simulink model "OnBoardMatlabExpo3"  (R2015b)
settings: Solver=FixedStepDiscrete  SolverMode=SingleTasking  StartTime=0.0  StopTime=10.0  FixedStep=0.002  RelTol=1e-3
PreLoadFcn:
  | waijung.modelPreload; % Required for working with Waijung Blockset. Do not remove.
undefined symbols (not defined in the file): CPHA_1Edge, CPOL_Low, Duplex, FirstBit_MSB, Full, Link, LQFP100, ST, STM32F407VG, STM32F4DISCOVERY
libraries: simulink x12, stm32f4_io_lib x7, cube_lib x3, stm32f4_spi_lib x3, stm32f4_device_config_lib x1, BC_USB x1, stm32f4_adc_lib x1
(part 2 of 2)

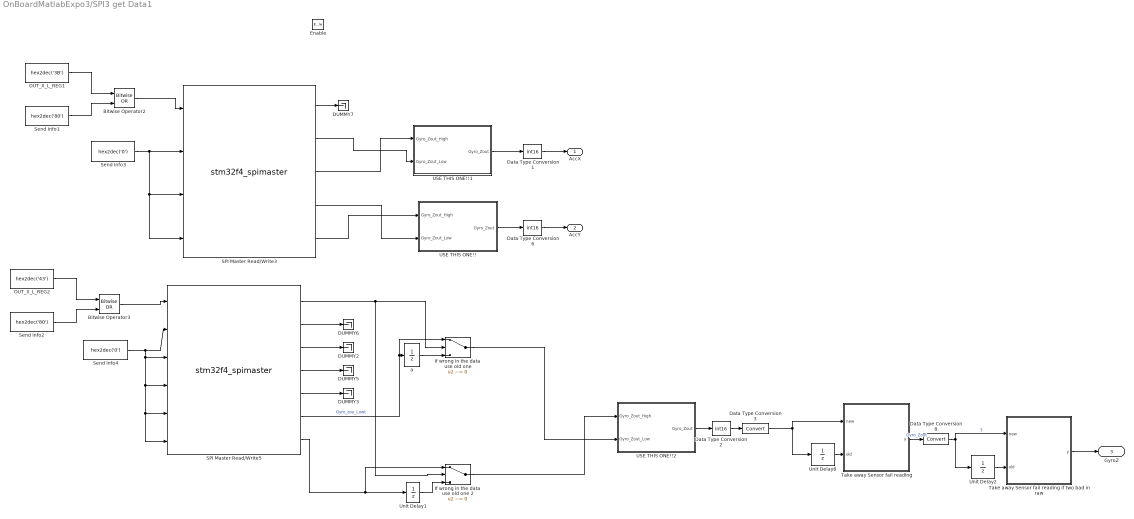
== system OnBoardMatlabExpo3/SPI3 get Data1 ==
  Enable : EnablePort
  " a" : UnitDelay  SampleTime=-1
  Bitwise Operator2 : simulink/Logic and Bit Operations/Bitwise Operator  logicop=OR  UseBitMask=off  NumInputPorts=2  BitMask=bin2dec('11011001')  BitMaskRealWorld=Stored Integer
  Bitwise Operator3 : simulink/Logic and Bit Operations/Bitwise Operator  logicop=OR  UseBitMask=off  NumInputPorts=2  BitMask=bin2dec('11011001')  BitMaskRealWorld=Stored Integer
  DUMMY{2..3,5..7} (5 alike) : Terminator
  Data Type Conversion1 : DataTypeConversion  OutDataTypeStr=int16
  Data Type Conversion2 : DataTypeConversion  OutDataTypeStr=int16
  Data Type Conversion3 : DataTypeConversion
  Data Type Conversion6 : DataTypeConversion  OutDataTypeStr=int16
  Data Type Conversion8 : DataTypeConversion
  If wrong in the data use old one : Switch  Criteria=u2 ~= 0
  If wrong in the data use old one 2 : Switch  Criteria=u2 ~= 0
  OUT_X_L_REG1 : Constant  Value=hex2dec('3B')  OutDataTypeStr=uint8
  OUT_X_L_REG2 : Constant  Value=hex2dec('43')  OutDataTypeStr=uint8
  SPI Master Read/Write3 : S-Function  FunctionName=stm32f4_spimaster  Parameters=mode,configuration,module,datacount,inputtypearray,outputtypearray,confstr,sampletime,sampletimestr,blockid  SFunctionDeploymentMode=off  EnableBusSupport=off  mask(stm32f4_spimaster){configuration=Transaction, module=3, mode=Read/ Write, lastmodule=1, direction=Full-Duplex, dataformat=8bit/ FirstBit_MSB, prescaler=4, cpolcpha=CPOL_Low/ CPHA_1Edge, datacount=4, nssmode=Custom, nsspin=Not used, softnssport=E, softnsspin=0, sckpin=A5, misopin=A6, mosipin=A7, inputtypearray=[4 3 3 3 3], outputtypearray=[5 7 3 3 3 3], confstr=["SPI_Direction_2Lines_FullDuplex","8b","MSB","Low","1Edge","4","Soft","0","x","x","0","x","x","1","A","5","1","A","6","1","A","7","1","0","0","0","0","0","0","0","0","PP","0","UP"], sampletime=-1, sampletimestr=Inf, blockid=SPI3getData1SPIMasterReadWrite3}
      mask prompts: module "SPI Module:"; lastmodule "Last module:"; dataformat "Data format:"; prescaler "Buad rate prescaler: Pclk/"; cpolcpha "Clock polarity (CPOL)/ Clock phase (CPHA):"; datacount "Data Read/Write count:"; nssmode "Slave/chip select (nSS, nCS) mode"; nsspin "Slave/chip select (nSS, nCS) pin"; softnssport "Slave/chip select port (nSS, nCS)"; softnsspin "Slave/chip select pin (nSS, nCS)"; sckpin "SCLK pin:"; misopin "MISO pin:"; mosipin "MOSI pin:"; inputtypearray "Input type array"; outputtypearray "Output type array"; confstr "Configuration string"; sampletime "Sample time (sec)"; sampletimestr "Compiled sample time (sec) in string"
      mask help:
      | Status:
      |  0 - Success.
      |  Otherwise - Fail.
      mask init:
      | stm32f4_spimaster_callback('init');
      mask Help: web(fullfile(waijungdocroot,'stm32f4_spimaster_readwrite.htm'), '-browser')
      mask TypeOptions configuration: Setup | Transaction
      mask Callback configuration: stm32f4_spimaster_callback('configuration');
      mask TypeOptions module: 1 | 2 | 3
      mask Callback module: stm32f4_spimaster_callback('module');
      mask TypeOptions mode: Read/ Write | Read | Write
      mask Callback mode: stm32f4_spimaster_callback('mode');
      mask TypeOptions direction: Full-Duplex | Half-Duplex_Tx | Half-Duplex_Rx
      mask Callback direction: stm32f4_spimaster_callback('direction');
      mask TypeOptions dataformat: 8bit/ FirstBit_MSB | 8bit/ FirstBit_LSB | 16bit/ FirstBit_MSB | 16bit/ FirstBit_LSB
      mask TypeOptions prescaler: 2 | 4 | 8 | 16 | 32 | 64 | 128 | 256
      mask TypeOptions cpolcpha: CPOL_Low/ CPHA_1Edge | CPOL_Low/ CPHA_2Edge | CPOL_High/ CPHA_1Edge | CPOL_High/ CPHA_2Edge
      mask Callback datacount: stm32f4_spimaster_callback('datacount');
      mask TypeOptions nssmode: Hardware | Software | Custom
      mask Callback nssmode: stm32f4_spimaster_callback('nssmode');
      mask TypeOptions nsspin: Not used | A4 | A15
      mask TypeOptions softnssport: A | B | C | D | E | F | G | H | I
      mask TypeOptions softnsspin: 0 | 1 | 2 | 3 | 4 | 5 | 6 | 7 | 8 | 9 | 10 | 11 | 12 | 13 | 14 | 15
      mask TypeOptions sckpin: Not used | A5 | B3
      mask TypeOptions misopin: Not used | A6 | B4
      mask TypeOptions mosipin: Not used | A7 | B5
      mask Callback confstr: stm32f4_spimaster_callback('confstr');
      mask Callback sampletime: stm32f4_spimaster_callback('sampletime');
      mask Callback sampletimestr: stm32f4_spimaster_callback('sampletimestr');
      mask Callback blockid: stm32f4_spimaster_callback('blockid');
      mask Display: text(0.5, 0.5, 'Module: SPI3 (Master)\nRead/ Write\nTs (sec): Inf','ver','middle','hor','center');port_label('input', 1,'Wr0 (uint8)');port_label('input', 2,'Wr1 (uint8)');port_label('input', 3,'Wr2 (uint8)');port_label('input', 4,'Wr3 (uint8)');port_label('output', 1,'Status');port_label('output', 2,'Rd0 (uint8)');port_label('output', 3,'Rd1 (uint8)');port_label('output', 4,'Rd2 (uint8)');port_label('output', 5,'Rd3 (uint8)');
  SPI Master Read/Write5 : S-Function  FunctionName=stm32f4_spimaster  Parameters=mode,configuration,module,datacount,inputtypearray,outputtypearray,confstr,sampletime,sampletimestr,blockid  SFunctionDeploymentMode=off  EnableBusSupport=off  mask(stm32f4_spimaster){configuration=Transaction, module=3, mode=Read/ Write, lastmodule=1, direction=Full-Duplex, dataformat=8bit/ FirstBit_MSB, prescaler=4, cpolcpha=CPOL_Low/ CPHA_1Edge, datacount=6, nssmode=Custom, nsspin=Not used, softnssport=E, softnsspin=0, sckpin=A5, misopin=A6, mosipin=A7, inputtypearray=[6 3 3 3 3 3 3], outputtypearray=[7 7 3 3 3 3 3 3], confstr=["SPI_Direction_2Lines_FullDuplex","8b","MSB","Low","1Edge","4","Soft","0","x","x","0","x","x","1","A","5","1","A","6","1","A","7","1","0","0","0","0","0","0","0","0","PP","0","UP"], sampletime=-1, sampletimestr=Inf, blockid=SPI3getData1SPIMasterReadWrite5}
      mask prompts: module "SPI Module:"; lastmodule "Last module:"; dataformat "Data format:"; prescaler "Buad rate prescaler: Pclk/"; cpolcpha "Clock polarity (CPOL)/ Clock phase (CPHA):"; datacount "Data Read/Write count:"; nssmode "Slave/chip select (nSS, nCS) mode"; nsspin "Slave/chip select (nSS, nCS) pin"; softnssport "Slave/chip select port (nSS, nCS)"; softnsspin "Slave/chip select pin (nSS, nCS)"; sckpin "SCLK pin:"; misopin "MISO pin:"; mosipin "MOSI pin:"; inputtypearray "Input type array"; outputtypearray "Output type array"; confstr "Configuration string"; sampletime "Sample time (sec)"; sampletimestr "Compiled sample time (sec) in string"
      mask help:
      | Status:
      |  0 - Success.
      |  Otherwise - Fail.
      mask init:
      | stm32f4_spimaster_callback('init');
      mask Help: web(fullfile(waijungdocroot,'stm32f4_spimaster_readwrite.htm'), '-browser')
      mask TypeOptions configuration: Setup | Transaction
      mask Callback configuration: stm32f4_spimaster_callback('configuration');
      mask TypeOptions module: 1 | 2 | 3
      mask Callback module: stm32f4_spimaster_callback('module');
      mask TypeOptions mode: Read/ Write | Read | Write
      mask Callback mode: stm32f4_spimaster_callback('mode');
      mask TypeOptions direction: Full-Duplex | Half-Duplex_Tx | Half-Duplex_Rx
      mask Callback direction: stm32f4_spimaster_callback('direction');
      mask TypeOptions dataformat: 8bit/ FirstBit_MSB | 8bit/ FirstBit_LSB | 16bit/ FirstBit_MSB | 16bit/ FirstBit_LSB
      mask TypeOptions prescaler: 2 | 4 | 8 | 16 | 32 | 64 | 128 | 256
      mask TypeOptions cpolcpha: CPOL_Low/ CPHA_1Edge | CPOL_Low/ CPHA_2Edge | CPOL_High/ CPHA_1Edge | CPOL_High/ CPHA_2Edge
      mask Callback datacount: stm32f4_spimaster_callback('datacount');
      mask TypeOptions nssmode: Hardware | Software | Custom
      mask Callback nssmode: stm32f4_spimaster_callback('nssmode');
      mask TypeOptions nsspin: Not used | A4 | A15
      mask TypeOptions softnssport: A | B | C | D | E | F | G | H | I
      mask TypeOptions softnsspin: 0 | 1 | 2 | 3 | 4 | 5 | 6 | 7 | 8 | 9 | 10 | 11 | 12 | 13 | 14 | 15
      mask TypeOptions sckpin: Not used | A5 | B3
      mask TypeOptions misopin: Not used | A6 | B4
      mask TypeOptions mosipin: Not used | A7 | B5
      mask Callback confstr: stm32f4_spimaster_callback('confstr');
      mask Callback sampletime: stm32f4_spimaster_callback('sampletime');
      mask Callback sampletimestr: stm32f4_spimaster_callback('sampletimestr');
      mask Callback blockid: stm32f4_spimaster_callback('blockid');
      mask Display: text(0.5, 0.5, 'Module: SPI3 (Master)\nRead/ Write\nTs (sec): Inf','ver','middle','hor','center');port_label('input', 1,'Wr0 (uint8)');port_label('input', 2,'Wr1 (uint8)');port_label('input', 3,'Wr2 (uint8)');port_label('input', 4,'Wr3 (uint8)');port_label('input', 5,'Wr4 (uint8)');port_label('input', 6,'Wr5 (uint8)');port_label('output', 1,'Status');port_label('output', 2,'Rd0 (uint8)');port_label('output', 3,'Rd1 (uint8)');port_label('output', 4,'Rd2 (uint8)');port_label('output', 5,'Rd3 (uint8)');port_label('output', 6,'Rd4 (uint8)');port_label('output', 7,'Rd5 (uint8)');
  Send Info1 : Constant  Value=hex2dec('80')  OutDataTypeStr=uint8
  Send Info2 : Constant  Value=hex2dec('80')  OutDataTypeStr=uint8
  Send Info3 : Constant  Value=hex2dec('0')  OutDataTypeStr=uint8
  Send Info4 : Constant  Value=hex2dec('0')  OutDataTypeStr=uint8
  Take away Sensor fail reading : MATLAB Function  TreatAsAtomicUnit=on
  Take away Sensor fail reading if two bad in raw : MATLAB Function  TreatAsAtomicUnit=on
  USE THIS ONE!! : Subsystem
  USE THIS ONE!!1 : Subsystem
  USE THIS ONE!!2 : Subsystem
  Unit Delay1 : UnitDelay  SampleTime=-1
  Unit Delay2 : UnitDelay  InitialCondition=-40.45  SampleTime=-1
  Unit Delay8 : UnitDelay  InitialCondition=-40.45  SampleTime=-1
  AccX : Outport
  "AccY " : Outport  Port=2
  GyroZ : Outport  Port=3
  wires:
  SPI Master Read/Write5/2 -> DUMMY6/1
  SPI Master Read/Write5/4 -> DUMMY5/1
  Bitwise Operator3/1 -> SPI Master Read/Write5/1
  OUT_X_L_REG1/1 -> Bitwise Operator2/1
  OUT_X_L_REG2/1 -> Bitwise Operator3/1
  Send Info2/1 -> Bitwise Operator3/2
  Bitwise Operator2/1 -> SPI Master Read/Write3/1
  Send Info3/1 -> SPI Master Read/Write3/4, SPI Master Read/Write3/3, SPI Master Read/Write3/2
  Send Info1/1 -> Bitwise Operator2/2
  Send Info4/1 -> SPI Master Read/Write5/6, SPI Master Read/Write5/5, SPI Master Read/Write5/4, SPI Master Read/Write5/3, SPI Master Read/Write5/2
  SPI Master Read/Write3/1 -> DUMMY7/1
  SPI Master Read/Write5/3 -> DUMMY2/1
  SPI Master Read/Write5/5 -> DUMMY3/1
  SPI Master Read/Write3/2 -> USE THIS ONE!!1/2(Gyro_Zout_Low)
  SPI Master Read/Write3/3 -> USE THIS ONE!!1/1("Gyro_Zout_High ")
  SPI Master Read/Write3/4 -> USE THIS ONE!!/2(Gyro_Zout_Low)
  SPI Master Read/Write3/5 -> USE THIS ONE!!/1("Gyro_Zout_High ")
  USE THIS ONE!!1/1(Gyro_Zout) -> Data Type Conversion1/1
  USE THIS ONE!!/1(Gyro_Zout) -> Data Type Conversion6/1
  Data Type Conversion6/1 -> "AccY "/1
  Data Type Conversion1/1 -> AccX/1
  USE THIS ONE!!2/1(Gyro_Zout) -> Data Type Conversion2/1
  Data Type Conversion2/1 -> Data Type Conversion3/1
  SPI Master Read/Write5/6 -> " a"/1, If wrong in the data use old one/1  "Gyro_zou_Lowt"
  " a"/1 -> If wrong in the data use old one/3
  SPI Master Read/Write5/7 -> If wrong in the data use old one 2/1, Unit Delay1/1
  SPI Master Read/Write5/1 -> If wrong in the data use old one 2/2, If wrong in the data use old one/2
  Unit Delay1/1 -> If wrong in the data use old one 2/3
  If wrong in the data use old one/1 -> USE THIS ONE!!2/2(Gyro_Zout_Low)
  If wrong in the data use old one 2/1 -> USE THIS ONE!!2/1("Gyro_Zout_High ")
  Unit Delay8/1 -> Take away Sensor fail reading/2(old)
  Take away Sensor fail reading/1(y) -> Data Type Conversion8/1  "Gyro_Zout"
  Unit Delay2/1 -> Take away Sensor fail reading if two bad in raw/2(old)
  Data Type Conversion8/1 -> Unit Delay2/1, Take away Sensor fail reading if two bad in raw/1(new)  "3"
  Take away Sensor fail reading if two bad in raw/1(y) -> GyroZ/1
  Data Type Conversion3/1 -> Unit Delay8/1, Take away Sensor fail reading/1(new)

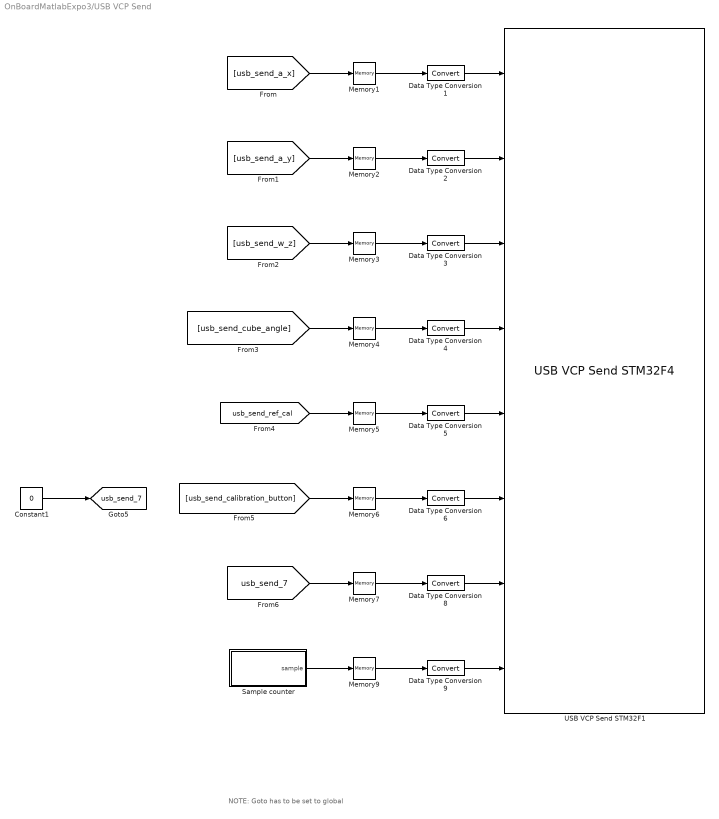
== system OnBoardMatlabExpo3/USB VCP Send ==
  note: NOTE: Goto has to be set to global
  Constant1 : Constant  Value=0
  Data Type Conversion{1..6,8..9} (8 alike) : DataTypeConversion
  Memory{1..7,9} (8 alike) : Memory  InheritSampleTime=on
  Sample counter : MATLAB Function  TreatAsAtomicUnit=on
  USB VCP Send STM32F1 : BC_USB/USB VCP Send STM32F4  speed="USB 1.1   12Mbit/s"  data_size=2048 Bytes  header_data='0E 0E'  binary_data='double double double double double double double double'  terminator_data='0A 0A'  sampletime=0.002
  tag scope: usb_send_7=global
  wires:
  Data Type Conversion2/1 -> USB VCP Send STM32F1/2
  Memory4/1 -> Data Type Conversion4/1
  [usb_send_ref_cal] -> Memory5/1
  Data Type Conversion8/1 -> USB VCP Send STM32F1/7
  Memory2/1 -> Data Type Conversion2/1
  Constant1/1 -> [usb_send_7]
  Memory5/1 -> Data Type Conversion5/1
  Memory1/1 -> Data Type Conversion1/1
  Data Type Conversion5/1 -> USB VCP Send STM32F1/5
  Memory9/1 -> Data Type Conversion9/1
  Data Type Conversion3/1 -> USB VCP Send STM32F1/3
  Data Type Conversion4/1 -> USB VCP Send STM32F1/4
  Data Type Conversion9/1 -> USB VCP Send STM32F1/8
  Memory3/1 -> Data Type Conversion3/1
  Data Type Conversion6/1 -> USB VCP Send STM32F1/6
  [usb_send_a_x] -> Memory1/1
  [usb_send_w_z] -> Memory3/1
  [usb_send_calibration_button] -> Memory6/1
  Memory7/1 -> Data Type Conversion8/1
  Data Type Conversion1/1 -> USB VCP Send STM32F1/1
  Memory6/1 -> Data Type Conversion6/1
  Sample counter/1(sample) -> Memory9/1
  [usb_send_cube_angle] -> Memory4/1
  [usb_send_7] -> Memory7/1
  [usb_send_a_y] -> Memory2/1

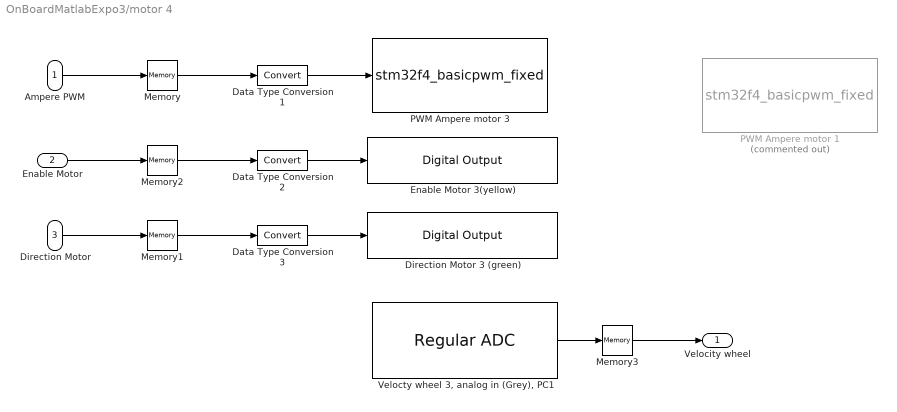
== system OnBoardMatlabExpo3/motor 4 ==
  Ampere PWM : Inport
  Enable Motor : Inport  Port=2
  "Direction Motor " : Inport  Port=3
  Data Type Conversion1 : DataTypeConversion
  Data Type Conversion2 : DataTypeConversion
  Data Type Conversion3 : DataTypeConversion
  Direction Motor 3 (green) : stm32f4_io_lib/Digital Output  use_bitband=on  port=D  speed=100  porttype=Push Pull  porttypestr=PP  use_pin0=off  use_pin1=off  use_pin2=off  use_pin3=off  use_pin4=off  use_pin5=off  use_pin6=off  use_pin7=off  use_pin8=off  use_pin9=off  use_pin10=off  use_pin11=on  use_pin12=off  use_pin13=off  use_pin14=off  use_pin15=off  pinstr=GPIO_Pin_11  usedpinarray="[0  0  0  0  0  0  0  0  0  0  0  1  0  0  0  0]"  bitbandingstr="#define motor4DirectionMotor3green_D11 Peripheral_BB(GPIOD->ODR, 11)  /* Output pin */"  sampletime=-1  sampletimestr=0.002  blockid=motor4DirectionMotor3green  enablecustomportlabel=off  globalinit=off  cinputportlabel=In1, In2  coutputportlabel=0
  Enable Motor 3(yellow) : stm32f4_io_lib/Digital Output  use_bitband=on  port=D  speed=100  porttype=Push Pull  porttypestr=PP  use_pin0=off  use_pin1=off  use_pin2=off  use_pin3=off  use_pin4=off  use_pin5=off  use_pin6=off  use_pin7=off  use_pin8=off  use_pin9=on  use_pin10=off  use_pin11=off  use_pin12=off  use_pin13=off  use_pin14=off  use_pin15=off  pinstr=GPIO_Pin_9  usedpinarray="[0  0  0  0  0  0  0  0  0  1  0  0  0  0  0  0]"  bitbandingstr="#define motor4EnableMotor3yellow_D9 Peripheral_BB(GPIOD->ODR, 9)  /* Output pin */"  sampletime=-1  sampletimestr=0.002  blockid=motor4EnableMotor3yellow  enablecustomportlabel=off  globalinit=off  cinputportlabel=In1, In2  coutputportlabel=0
  Memory{,1..3} (4 alike) : Memory  InheritSampleTime=on
  PWM Ampere motor 1 : S-Function  Commented=on  FunctionName=stm32f4_basicpwm_fixed  Parameters=timer,pwmperiod,uc3m_pwmperiod,ch1pin,ch2pin,ch3pin,ch4pin,sampletime,sampletimestr,blockid,apb,portstr,pinstr,pinmat,timarr,timprescale,chmat,polaritystr  SFunctionDeploymentMode=off  EnableBusSupport=off  mask(stm32f4_basicpwm_fixed){timer=5, pwmperiod=0.02, uc3m_pwmperiod=0.0002, polarity=Active High, polaritystr=TIM_OCPolarity_High, ch1pin=Not available - Do not use, ch2pin=Not available - Do not use, ch3pin=Not available - Do not use, ch4pin=A3, sampletime=0.002, sampletimestr=0.002, blockid=motor3PWMAmperemotor3, portpinstr=,,,A3, enablecustomportlabel=off, cinputportlabel=In1, In2, In3, In4, coutputportlabel=0, callbackgensrccode=off, apb=1, portstr=["A"], pinstr=["GPIO_Pin_3"], pinmat=[1 3], timarr=59999, timprescale=55, chmat=[4]}
      mask prompts: pwmperiod "PWM Period (seconds)"; uc3m_pwmperiod "PWM Signal Period (seconds)"; ch1pin "Channel 1"; ch2pin "Channel 2"; ch3pin "Channel 3"; ch4pin "Channel 4"; sampletime "Sample time (sec)"; sampletimestr "Compiled sample time (sec) in string"; portpinstr "Port pin string"; enablecustomportlabel "Enable custom port labels"; cinputportlabel "Custom input port labels (Ex. In1, In2, In3)"; coutputportlabel "Custom output port labels (Ex. Out1, Out2, Out3)"; callbackgensrccode "Gen source code from callback"; portstr "Port string"; pinstr "Pin string"; pinmat "Pin matrix"; timarr "Timer ARR"; timprescale "Timer PRESCALE"; chmat "Channel order"
      mask help:
      | This block implements basic Edge-aligned Pulse Width Modulation (PWM) generation.
      | All timers are 16-bit. The PWM period is fixed (per timer).
      |
      | This block was fixed by Sr Antonio
      mask init:
      | stm32f4_basicpwm_callback_fixed('init');
      mask Help: web(fullfile(waijungdocroot,'stm32f4_basicpwm.htm'),'-browser')
      mask TypeOptions timer: 1 | 2 | 3 | 4 | 5 | 8 | 9 | 10 | 11 | 12 | 13 | 14
      mask Callback timer: stm32f4_basicpwm_callback_fixed('timer');
      mask Callback pwmperiod: stm32f4_basicpwm_callback_fixed('pwmperiod');
      mask Callback uc3m_pwmperiod: stm32f4_basicpwm_callback_fixed('uc3m_pwmperiod');
      mask TypeOptions polarity: Active High | Active Low
      mask Callback polarity: stm32f4_basicpwm_callback_fixed('polarity');
      mask TypeOptions ch1pin: Not available - Do not use | A0 | A5
      mask Callback ch1pin: stm32f4_basicpwm_callback_fixed('ch1pin');
      mask TypeOptions ch2pin: Not available - Do not use | A1 | B3
      mask Callback ch2pin: stm32f4_basicpwm_callback_fixed('ch2pin');
      mask TypeOptions ch3pin: Not available - Do not use | A2 | B10
      mask Callback ch3pin: stm32f4_basicpwm_callback_fixed('ch3pin');
      mask TypeOptions ch4pin: Not available - Do not use | A3 | B11
      mask Callback ch4pin: stm32f4_basicpwm_callback_fixed('ch4pin');
      mask Callback sampletime: stm32f4_basicpwm_callback_fixed('sampletime');
      mask Callback sampletimestr: stm32f4_basicpwm_callback_fixed('sampletimestr');
      mask Callback blockid: stm32f4_basicpwm_callback_fixed('blockid');
      mask Callback enablecustomportlabel: stm32f4_basicpwm_callback_fixed('enablecustomportlabel')
      mask Display: text(0.95, 0.5, 'UC3M FIXED\nTimer: 5\nPolarity: Active High\nPeriod (sec): 0.0002\nTs (sec): 0.002','ver','middle','hor','right');port_label('input', 1,'CH4 (A3)')
  PWM Ampere motor 3 : S-Function  FunctionName=stm32f4_basicpwm_fixed  Parameters=timer,pwmperiod,uc3m_pwmperiod,ch1pin,ch2pin,ch3pin,ch4pin,sampletime,sampletimestr,blockid,apb,portstr,pinstr,pinmat,timarr,timprescale,chmat,polaritystr  SFunctionDeploymentMode=off  EnableBusSupport=off  mask(stm32f4_basicpwm_fixed){timer=2, pwmperiod=0.02, uc3m_pwmperiod=0.0002, polarity=Active High, polaritystr=TIM_OCPolarity_High, ch1pin=Not available - Do not use, ch2pin=Not available - Do not use, ch3pin=Not available - Do not use, ch4pin=A3, sampletime=0.002, sampletimestr=0.002, blockid=motor4PWMAmperemotor3, portpinstr=,,,A3, enablecustomportlabel=off, cinputportlabel=In1, In2, In3, In4, coutputportlabel=0, callbackgensrccode=off, apb=1, portstr=["A"], pinstr=["GPIO_Pin_3"], pinmat=[1 3], timarr=59999, timprescale=55, chmat=[4]}
      mask prompts: pwmperiod "PWM Period (seconds)"; uc3m_pwmperiod "PWM Signal Period (seconds)"; ch1pin "Channel 1"; ch2pin "Channel 2"; ch3pin "Channel 3"; ch4pin "Channel 4"; sampletime "Sample time (sec)"; sampletimestr "Compiled sample time (sec) in string"; portpinstr "Port pin string"; enablecustomportlabel "Enable custom port labels"; cinputportlabel "Custom input port labels (Ex. In1, In2, In3)"; coutputportlabel "Custom output port labels (Ex. Out1, Out2, Out3)"; callbackgensrccode "Gen source code from callback"; portstr "Port string"; pinstr "Pin string"; pinmat "Pin matrix"; timarr "Timer ARR"; timprescale "Timer PRESCALE"; chmat "Channel order"
      mask help:
      | This block implements basic Edge-aligned Pulse Width Modulation (PWM) generation.
      | All timers are 16-bit. The PWM period is fixed (per timer).
      |
      | This block was fixed by Sr Antonio
      mask init:
      | stm32f4_basicpwm_callback_fixed('init');
      mask Help: web(fullfile(waijungdocroot,'stm32f4_basicpwm.htm'),'-browser')
      mask TypeOptions timer: 1 | 2 | 3 | 4 | 5 | 8 | 9 | 10 | 11 | 12 | 13 | 14
      mask Callback timer: stm32f4_basicpwm_callback_fixed('timer');
      mask Callback pwmperiod: stm32f4_basicpwm_callback_fixed('pwmperiod');
      mask Callback uc3m_pwmperiod: stm32f4_basicpwm_callback_fixed('uc3m_pwmperiod');
      mask TypeOptions polarity: Active High | Active Low
      mask Callback polarity: stm32f4_basicpwm_callback_fixed('polarity');
      mask TypeOptions ch1pin: Not available - Do not use | A0 | A5
      mask Callback ch1pin: stm32f4_basicpwm_callback_fixed('ch1pin');
      mask TypeOptions ch2pin: Not available - Do not use | A1 | B3
      mask Callback ch2pin: stm32f4_basicpwm_callback_fixed('ch2pin');
      mask TypeOptions ch3pin: Not available - Do not use | A2 | B10
      mask Callback ch3pin: stm32f4_basicpwm_callback_fixed('ch3pin');
      mask TypeOptions ch4pin: Not available - Do not use | A3 | B11
      mask Callback ch4pin: stm32f4_basicpwm_callback_fixed('ch4pin');
      mask Callback sampletime: stm32f4_basicpwm_callback_fixed('sampletime');
      mask Callback sampletimestr: stm32f4_basicpwm_callback_fixed('sampletimestr');
      mask Callback blockid: stm32f4_basicpwm_callback_fixed('blockid');
      mask Callback enablecustomportlabel: stm32f4_basicpwm_callback_fixed('enablecustomportlabel')
      mask Display: text(0.95, 0.5, 'UC3M FIXED\nTimer: 2\nPolarity: Active High\nPeriod (sec): 0.0002\nTs (sec): 0.002','ver','middle','hor','right');port_label('input', 1,'CH4 (A3)')
  "Velocty wheel 3, analog in (Grey), PC1" : stm32f4_adc_lib/Regular ADC  adcmodule=3  outputdatatype=Double  prescaler=2  prescalerstr=ADC_Prescaler_Div2  chsamplingtime=Auto  chsamplingtimestr=ADC_SampleTime_480Cycles  read_an0=off  read_an1=off  read_an2=off  read_an3=off  read_an4=off  read_an5=off  read_an6=off  read_an7=off  read_an8=off  read_an9=off  read_an10=off  read_an11=on  read_an12=off  read_an13=off  read_an14=off  read_an15=off  read_an16=off  read_an17=off  read_an18=off  pinstr=GPIO_Pin_11  usedpinarray="[0  0  0  0  0  0  0  0  0  0  0  1  0  0  0  0  0  0  0]"  usedportidarray=[2]  usedpinidarray=[1]  usedpinidcount=1  sampletime=0.002  blockid=motor4Veloctywheel3analoginGreyPC1  enablecustomportlabel=off  cinputportlabel=0  coutputportlabel=Out1, Out2
  Velocity wheel : Outport
  wires:
  Ampere PWM/1 -> Memory/1
  Data Type Conversion3/1 -> Direction Motor 3 (green)/1
  Data Type Conversion2/1 -> Enable Motor 3(yellow)/1
  Memory/1 -> Data Type Conversion1/1
  Memory2/1 -> Data Type Conversion2/1
  "Direction Motor "/1 -> Memory1/1
  Memory1/1 -> Data Type Conversion3/1
  Enable Motor/1 -> Memory2/1
  "Velocty wheel 3, analog in (Grey), PC1"/1 -> Memory3/1
  Memory3/1 -> Velocity wheel/1
  Data Type Conversion1/1 -> PWM Ampere motor 3/1

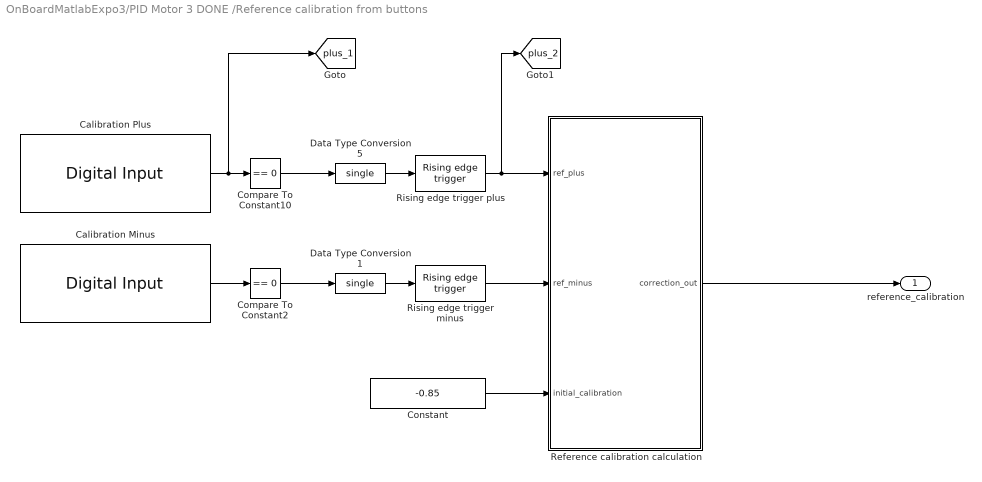
== system OnBoardMatlabExpo3/PID Motor 3 DONE /Reference calibration from buttons ==
  Calibration Minus : stm32f4_io_lib/Digital Input  port=E  speed=100  porttype=Pull Up  porttypestr=UP  use_pin0=off  use_pin1=off  use_pin2=off  use_pin3=off  use_pin4=off  use_pin5=off  use_pin6=off  use_pin7=off  use_pin8=off  use_pin9=off  use_pin10=off  use_pin11=off  use_pin12=off  use_pin13=off  use_pin14=on  use_pin15=off  pinstr=GPIO_Pin_14  usedpinarray="[0  0  0  0  0  0  0  0  0  0  0  0  0  0  1  0]"  bitbandingstr="#define PIDMotor3DONEReferencecalibrationfrombuttonsCalibrationMinus_E14 Peripheral_BB(GPIOE->IDR, 14)  /* Output pin */"  sampletime=0.002  sampletimestr=0.002  blockid=PIDMotor3DONEReferencecalibrationfrombuttonsCalibrationMinus  enablecustomportlabel=off  glabalinit=off  cinputportlabel=In1, In2  coutputportlabel=Out1, Out2
  Calibration Plus : stm32f4_io_lib/Digital Input  port=E  speed=100  porttype=Pull Up  porttypestr=UP  use_pin0=off  use_pin1=off  use_pin2=off  use_pin3=off  use_pin4=off  use_pin5=off  use_pin6=off  use_pin7=off  use_pin8=off  use_pin9=off  use_pin10=off  use_pin11=on  use_pin12=off  use_pin13=off  use_pin14=off  use_pin15=off  pinstr=GPIO_Pin_11  usedpinarray="[0  0  0  0  0  0  0  0  0  0  0  1  0  0  0  0]"  bitbandingstr="#define PIDMotor3DONEReferencecalibrationfrombuttonsCalibrationPlus_E11 Peripheral_BB(GPIOE->IDR, 11)  /* Output pin */"  sampletime=0.002  sampletimestr=0.002  blockid=PIDMotor3DONEReferencecalibrationfrombuttonsCalibrationPlus  enablecustomportlabel=off  glabalinit=off  cinputportlabel=In1, In2  coutputportlabel=Out1, Out2
  Compare To Constant10 : simulink/Logic and Bit Operations/Compare To Constant  relop===  const=0  OutDataTypeStr=boolean  ZeroCross=off
  Compare To Constant2 : simulink/Logic and Bit Operations/Compare To Constant  relop===  const=0  OutDataTypeStr=boolean  ZeroCross=off
  Constant : Constant  Value=-0.85
  Data Type Conversion1 : DataTypeConversion  OutDataTypeStr=single
  Data Type Conversion5 : DataTypeConversion  OutDataTypeStr=single
  Reference calibration calculation : MATLAB Function  TreatAsAtomicUnit=on
  Rising edge trigger minus : cube_lib/Rising edge trigger
  Rising edge trigger plus : cube_lib/Rising edge trigger
  reference_calibration : Outport
  tag scope: plus_1=global, plus_2=global
  wires:
  Data Type Conversion5/1 -> Rising edge trigger plus/1
  Reference calibration calculation/1(correction_out) -> reference_calibration/1
  Calibration Minus/1 -> Compare To Constant2/1
  Compare To Constant10/1 -> Data Type Conversion5/1
  Compare To Constant2/1 -> Data Type Conversion1/1
  Calibration Plus/1 -> [plus_1], Compare To Constant10/1
  Rising edge trigger minus/1 -> Reference calibration calculation/2(ref_minus)
  Data Type Conversion1/1 -> Rising edge trigger minus/1
  Rising edge trigger plus/1 -> [plus_2], Reference calibration calculation/1(ref_plus)
  Constant/1 -> Reference calibration calculation/3(initial_calibration)

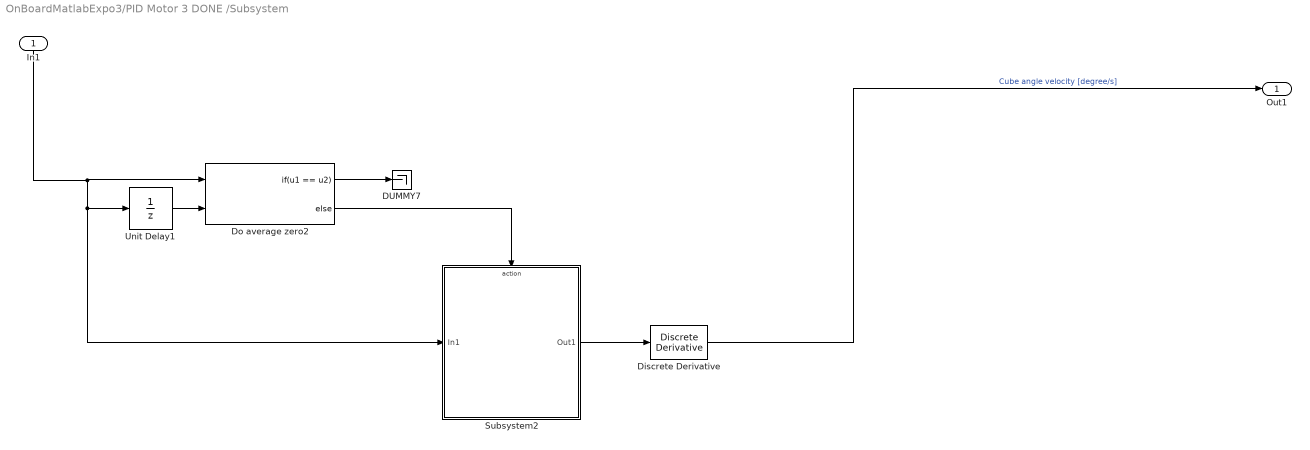
== system OnBoardMatlabExpo3/PID Motor 3 DONE /Subsystem ==
  In1 : Inport
  DUMMY7 : Terminator
  Discrete Derivative : simulink/Discrete/Discrete Derivative  gainval=1.0  ICPrevScaledInput=0.0  InputProcessing=Inherited  OutMin=[]  OutMax=[]  OutDataType=fixdt(1, 16)  OutScaling=2^-10  DoSatur=off
  Do average zero2 : If  NumInputs=2  IfExpression=u1 == u2
  Subsystem2 : Subsystem
  Unit Delay1 : UnitDelay  SampleTime=-1
  Out1 : Outport
  wires:
  Do average zero2/2 -> Subsystem2/Action
  Unit Delay1/1 -> Do average zero2/2
  Discrete Derivative/1 -> Out1/1  "Cube angle velocity [degree/s]"
  Subsystem2/1(Out1) -> Discrete Derivative/1
  In1/1 -> Subsystem2/1(In1), Unit Delay1/1, Do average zero2/1
  Do average zero2/1 -> DUMMY7/1

== system OnBoardMatlabExpo3/PID Motor 3 DONE /Subsystem2 ==
  In1 : Inport
  DUMMY7 : Terminator
  Do average zero1 : If  NumInputs=2  IfExpression=u1 == u2
  Subsystem1 : Subsystem
  Unit Delay3 : UnitDelay  SampleTime=-1
  Out2 : Outport
  wires:
  Unit Delay3/1 -> Do average zero1/2
  Do average zero1/2 -> Subsystem1/Action
  In1/1 -> Subsystem1/1(In1), Unit Delay3/1, Do average zero1/1
  Subsystem1/1(Out1) -> Out2/1
  Do average zero1/1 -> DUMMY7/1

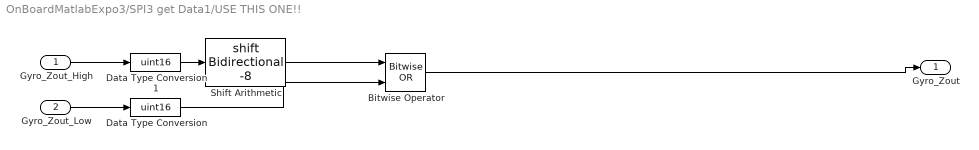
== system OnBoardMatlabExpo3/SPI3 get Data1/USE THIS ONE!! ==
  "Gyro_Zout_High " : Inport
  Gyro_Zout_Low : Inport  Port=2
  Bitwise Operator : simulink/Logic and Bit Operations/Bitwise Operator  logicop=OR  UseBitMask=off  NumInputPorts=2  BitMask=bin2dec('11011001')  BitMaskRealWorld=Stored Integer
  Data Type Conversion : DataTypeConversion  OutDataTypeStr=uint16
  Data Type Conversion1 : DataTypeConversion  OutDataTypeStr=uint16
  Shift Arithmetic : ArithShift  BitShiftNumber=-8
  Gyro_Zout : Outport
  wires:
  Gyro_Zout_Low/1 -> Data Type Conversion/1
  "Gyro_Zout_High "/1 -> Data Type Conversion1/1
  Data Type Conversion1/1 -> Shift Arithmetic/1
  Data Type Conversion/1 -> Bitwise Operator/2
  Shift Arithmetic/1 -> Bitwise Operator/1
  Bitwise Operator/1 -> Gyro_Zout/1

== system OnBoardMatlabExpo3/SPI3 get Data1/USE THIS ONE!!1 ==
  "Gyro_Zout_High " : Inport
  Gyro_Zout_Low : Inport  Port=2
  Bitwise Operator : simulink/Logic and Bit Operations/Bitwise Operator  logicop=OR  UseBitMask=off  NumInputPorts=2  BitMask=bin2dec('11011001')  BitMaskRealWorld=Stored Integer
  Data Type Conversion : DataTypeConversion  OutDataTypeStr=uint16
  Data Type Conversion1 : DataTypeConversion  OutDataTypeStr=uint16
  Shift Arithmetic : ArithShift  BitShiftNumber=-8
  Gyro_Zout : Outport
  wires:
  Gyro_Zout_Low/1 -> Data Type Conversion/1
  "Gyro_Zout_High "/1 -> Data Type Conversion1/1
  Data Type Conversion1/1 -> Shift Arithmetic/1
  Data Type Conversion/1 -> Bitwise Operator/2
  Shift Arithmetic/1 -> Bitwise Operator/1
  Bitwise Operator/1 -> Gyro_Zout/1

== system OnBoardMatlabExpo3/SPI3 get Data1/USE THIS ONE!!2 ==
  "Gyro_Zout_High " : Inport
  Gyro_Zout_Low : Inport  Port=2
  Bitwise Operator : simulink/Logic and Bit Operations/Bitwise Operator  logicop=OR  UseBitMask=off  NumInputPorts=2  BitMask=bin2dec('11011001')  BitMaskRealWorld=Stored Integer
  Data Type Conversion : DataTypeConversion  OutDataTypeStr=uint16
  Data Type Conversion1 : DataTypeConversion  OutDataTypeStr=uint16
  Shift Arithmetic : ArithShift  BitShiftNumber=-8
  Gyro_Zout : Outport
  wires:
  Gyro_Zout_Low/1 -> Data Type Conversion/1
  "Gyro_Zout_High "/1 -> Data Type Conversion1/1
  Data Type Conversion1/1 -> Shift Arithmetic/1
  Data Type Conversion/1 -> Bitwise Operator/2
  Shift Arithmetic/1 -> Bitwise Operator/1
  Bitwise Operator/1 -> Gyro_Zout/1

== system OnBoardMatlabExpo3/PID Motor 3 DONE /Subsystem/Subsystem2 ==
  In1 : Inport
  Action Port : ActionPort  ActionType=else
  Subsystem : Subsystem
  Unit Delay1 : UnitDelay  SampleTime=-1
  Out1 : Outport
  wires:
  In1/1 -> Subsystem/1(In1)
  Subsystem/1(Average Speed) -> Out1/1  "Speed, PA1"
  Subsystem/2(One old Speed) -> Unit Delay1/1
  Unit Delay1/1 -> Subsystem/2(One old speed)

== system OnBoardMatlabExpo3/PID Motor 3 DONE /Subsystem2/Subsystem1 ==
  In1 : Inport
  Action Port : ActionPort  ActionType=else
  Subsystem : Subsystem
  Unit Delay1 : UnitDelay  SampleTime=-1
  Out1 : Outport
  wires:
  In1/1 -> Subsystem/1(In1)
  Subsystem/1(Average Speed) -> Out1/1  "Speed, PA1"
  Subsystem/2(One old Speed) -> Unit Delay1/1
  Unit Delay1/1 -> Subsystem/2(One old speed)

== system OnBoardMatlabExpo3/PID Motor 3 DONE /Subsystem/Subsystem2/Subsystem ==
  In1 : Inport
  One old speed : Inport  Port=2
  Add2 : Sum
  Gain2 : Gain  Gain=0.5
  Gain3 : Gain  Gain=0.5
  Average Speed : Outport
  One old Speed : Outport  Port=2
  wires:
  Add2/1 -> One old Speed/1, Average Speed/1  "Speed, PA1"
  One old speed/1 -> Gain2/1
  In1/1 -> Gain3/1
  Gain2/1 -> Add2/2
  Gain3/1 -> Add2/1

== system OnBoardMatlabExpo3/PID Motor 3 DONE /Subsystem2/Subsystem1/Subsystem ==
  In1 : Inport
  One old speed : Inport  Port=2
  Add2 : Sum
  Gain2 : Gain  Gain=0.3
  Gain3 : Gain  Gain=0.7
  Average Speed : Outport
  One old Speed : Outport  Port=2
  wires:
  Add2/1 -> One old Speed/1, Average Speed/1  "Speed, PA1"
  One old speed/1 -> Gain2/1
  In1/1 -> Gain3/1
  Gain2/1 -> Add2/2
  Gain3/1 -> Add2/1

== matlab function OnBoardMatlabExpo3/PID Motor 3 DONE /Reference calibration from buttons/Reference calibration calculation ==
  data: ref_plus input; correction_out output; ref_minus input; initial_calibration input
function correction_out = ReferenceCalibration(ref_plus,ref_minus,initial_calibration)
%#codegen

persistent correction;

delta_correction = 0.05; % NOTE: Degrees!

if isempty(correction)
    correction = initial_calibration;   % Initial calibration is estimated center of gravity offset from geometrical center, in degrees.
end

if ref_plus == 1
    correction = correction + delta_correction;
end

if ref_minus == 1
    correction = correction - delta_correction;
end

correction_out = correction;

== matlab function OnBoardMatlabExpo3/Complementary filter system 2D 2 0 deg shift/Complementary filter ==
  data: a_x input size=1; a_y input size=1; w_z input size=1; misalignment input size=1; cube_angle output; errors_estimated input size=1
function cube_angle = ComplementaryFilter(a_x,a_y,w_z,misalignment,errors_estimated)
%#codegen
% Uses the equation:
% theta(k) = alfa*(theta(k-1) + w_z*T) + (1-alfa)*a(k);
% where a(k) is the estimated angle from the accelerometers
%
% alfa from cubeparameters

persistent theta_k_1; % Previous cube angle
persistent initiate_filter;

alfa = 0.995;
T_onboard = 0.002;
angle_correction = 135*pi/180; % Due to mounting

if isempty(theta_k_1)
    initiate_filter = 1;
    theta_k_1 = 0;
end

if errors_estimated && initiate_filter % First call to complementary filter (when no previous value exists)
    theta = atan2(a_x,a_y)-misalignment;
    initiate_filter = 0;
elseif errors_estimated
    % Complementary filter
    a_k = atan2(a_x,a_y)-misalignment; % Angle estimation from accelerometers
    % Improvement: Compensate for angular acceleration and centripetal
    % force
    theta = alfa*(theta_k_1 + w_z*T_onboard) + (1-alfa)*a_k;
else
    theta = 0;
end

theta_k_1 = theta;  % Save value

% Assign output
if errors_estimated
    cube_angle = theta + angle_correction;
else
    cube_angle = 0;
end

== matlab function OnBoardMatlabExpo3/Complementary filter system 2D 2 0 deg shift/Convert to SI units ==
  data: a_x input; a_x_data output double; a_y input; w_z input; a_y_data output double; w_z_data output double
function [a_x_data,a_y_data,w_z_data] = ConvertImuData(a_x,a_y,w_z)
%#codegen

g_ = 9.81*m_/s_^2;
a_scale_factor = 16384; % AFS_SEL = 0, se datablad MPU9250
w_scale_factor = 131;   % FS_SEL = 0, se datablad MPU9250
a_x_data = double(a_x)/a_scale_factor*g_;
a_y_data = double(a_y)/a_scale_factor*g_;
w_z_data = double(w_z)/w_scale_factor*deg_;

== matlab function OnBoardMatlabExpo3/Complementary filter system 2D 2 0 deg shift/Error estimation ==
  data: a_x input; a_x_corr output; a_y_corr output; w_z_corr output; misalignment_out output; a_y input; w_z input; state input; errors_estimated_out output
function [a_x_corr,a_y_corr,w_z_corr,misalignment_out,errors_estimated_out] = ErrorEstimatedImu(a_x,a_y,w_z,state)
%#codegen
% Finds IMU errors and corrects IMU data
persistent a_x_1; % Vector
persistent a_x_2; % Vector
persistent a_y_1; % Vector
persistent a_y_2; % Vector
persistent w_z_1; % Vector
persistent w_z_2; % Vector
persistent w_z_turn; % Scalar (sum)
persistent n_samples_w_z_turn; % Counts number of samples used for turn to compensate for bias
persistent k_sample;
persistent previous_state;
persistent errors_estimated;
persistent bias_a_x;
persistent bias_a_y;
persistent bias_w_z;
persistent scale_factor_a_x;
persistent scale_factor_a_y;
persistent scale_factor_w_z;
persistent misalignment;

n_samples = 1000; % Two seconds with T=0.002. Hardcoded for compiler
T_onboard = 0.002; % So that it does not have to be input or a set parameter

if isempty(a_x_1)
    k_sample = 1;
    previous_state = 0;
    errors_estimated = 0;
    a_x_1 = zeros(n_samples,1);
    a_x_2 = zeros(n_samples,1);
    a_y_1 = zeros(n_samples,1);
    a_y_2 = zeros(n_samples,1);
    w_z_1 = zeros(n_samples,1);
    w_z_2 = zeros(n_samples,1);
    w_z_turn = 0;
    n_samples_w_z_turn = 0;
    bias_a_x = 0;
    bias_a_y = 0;
    bias_w_z = 0;
    scale_factor_a_x = 0;
    scale_factor_a_y = 0;
    scale_factor_w_z = 0;
    misalignment = 0;
end

if state ~= previous_state % Entering a new state
    k_sample = 1;
    if state == 0 % Start over
        errors_estimated = 0;
        a_x_1 = zeros(n_samples,1);
        a_x_2 = zeros(n_samples,1);
        a_y_1 = zeros(n_samples,1);
        a_y_2 = zeros(n_samples,1);
        w_z_1 = zeros(n_samples,1);
        w_z_2 = zeros(n_samples,1);
        w_z_turn = 0;
        n_samples_w_z_turn = 0;
        bias_a_x = 0;
        bias_a_y = 0;
        bias_w_z = 0;
        scale_factor_a_x = 0;
        scale_factor_a_y = 0;
        scale_factor_w_z = 0;
        misalignment = 0;
    end
end

% Collect data in two phases, where cube_angle = -45 deg and cube_angle = 45 deg
if state == 1 && k_sample <= n_samples
    a_x_1(k_sample) = a_x;
    a_y_1(k_sample) = a_y;
    w_z_1(k_sample) = w_z;
    k_sample = k_sample + 1;
elseif state == 1
    w_z_turn = w_z_turn + w_z;
    n_samples_w_z_turn = n_samples_w_z_turn + 1;
    
end

if state == 2 && k_sample <= n_samples
    a_x_2(k_sample) = a_x;
    a_y_2(k_sample) = a_y;
    w_z_2(k_sample) = w_z;
    k_sample = k_sample + 1;
end

% Estimate errors when data from the two fixed positions have been done
if state == 2 && k_sample > n_samples && ~errors_estimated % We can estimate the errors
    % Sections
    a_x_1_meas = mean(a_x_1);
    a_x_2_meas = mean(a_x_2);
    a_y_1_meas = mean(a_y_1);
    a_y_2_meas = mean(a_y_2);
    w_z_meas   = mean([w_z_1;w_z_2]);
    
    % Call error estimation function
    % Derive expressions from this equations system:
    %  / a_1_measured = scale_factor*a_2_true + bias
    % {
    %  \ a_2_measured = scale_factor*a_2_true + bias
    g = 9.81;
    
    % IMU aligned with cube side, so that the y-axis points downwards when
    % the text MOTOR 3 is correctly horizontally aligned
    % First position:  a_x = 0, a_y = g
    % Second position: a_x = g, a_y = 0
    % That means:
    % a_x_1_meas = bias_x
    % a_x_2_meas = scale_factor_x*-g+bias_x = scale_factor_x*-g + a_x_1_meas
    %   and
    % a_y_1_meas = scale_factor_y*-g+bias_y = scale_factor_y*-g + a_y_1_meas
    % a_y_2_meas = bias_y
    % Great!
    bias_a_x = a_x_1_meas;
    bias_a_y = a_y_2_meas;
    scale_factor_a_x = (a_x_1_meas-a_x_2_meas)/g;
    scale_factor_a_y = (a_y_2_meas-a_y_1_meas)/g;
    
    % Gyro
    bias_w_z = w_z_meas; % Cube is still. What is measured is bias (and error)
    scale_factor_w_z = w_z_turn*T_onboard/(pi/2)-n_samples_w_z_turn*bias_w_z*T_onboard/(pi/2); % Should be a pi/2 turn. Compensate for bias.
    
    % Misalignment
    misalignment = 0;
    
    errors_estimated = 1;
end

% Update
previous_state = state;

% Assign output
if errors_estimated
    a_x_corr = (a_x-bias_a_x)/scale_factor_a_x;
    a_y_corr = (a_y-bias_a_y)/scale_factor_a_y;
    w_z_corr = (w_z-bias_w_z)/scale_factor_w_z;
else
    a_x_corr = a_x;
    a_y_corr = a_y;
    w_z_corr = w_z;
end

misalignment_out = misalignment;
errors_estimated_out = errors_estimated;

== matlab function OnBoardMatlabExpo3/Complementary filter system 2D 2 0 deg shift/State machine ==
  data: calibration_button input; state_out output
function state_out = StateMachine(calibration_button)
%#codegen
% Step between states 0, 1 and 2 from calibration button

persistent previous_value;
persistent sample;
persistent state;
persistent button_released;

min_samples_between_state_shift = 500; % 500 = 1 s

if isempty(previous_value)
    previous_value = false;
    state = 0;
    sample = min_samples_between_state_shift; % So that button can be clicked instantly
    button_released = true; % Button should be released inbetween clicks
end

if previous_value == 0 && calibration_button == 1 && sample > min_samples_between_state_shift && button_released
    state = state + 1;
    sample = 0;
    button_released = false;
end

if state == 3 % Start over
    state = 0;
end

if previous_value == 1 && calibration_button == 0
    button_released = true;
end

% Increment
sample = sample + 1;
previous_value = calibration_button;

% Assign output
state_out = state;

== matlab function OnBoardMatlabExpo3/Enabled Subsystem/Hold value ==
  data: u input; y output
function y = HoldValue(u)
%#codegen
% Holds high value for a number of samples
persistent sample;

n_samples_to_hold = 10;

if isempty(sample)
    sample = n_samples_to_hold;
end

if u == 1 || sample < n_samples_to_hold  % Only once per going high (trigged)
    y = 1;
    sample = sample - 1;
    if sample == 0
        sample = n_samples_to_hold;
    end
else
    y = 0;
end

== matlab function OnBoardMatlabExpo3/USB VCP Send/Sample counter ==
  data: sample output
function sample = SampleCounter
%#codegen

persistent sample_count;

if isempty(sample_count)
    sample_count = 0;
end

sample_count = sample_count + 1;

sample = sample_count;

== matlab function OnBoardMatlabExpo3/SPI3 get Data1/Take away Sensor fail reading ==
  data: y output; new input; old input
function y = fcn(new, old)
%#codegen
if(new > -257 && new < -200)
   y = old;
else
    y = new;
end

== matlab function OnBoardMatlabExpo3/SPI3 get Data1/Take away Sensor fail reading if two bad in raw ==
  data: y output; new input; old input
function y = fcn(new, old)
%#codegen
if(new > -257 && new < -200)
   y = old;
else
    y = new;
end
